simulink model "CalcTimes"  (R2024b)
settings: Solver=VariableStepAuto  StartTime=0.0  StopTime=10.0  RelTol=1e-3
settings Model: Creator=CArias  LastModifiedBy=CArias

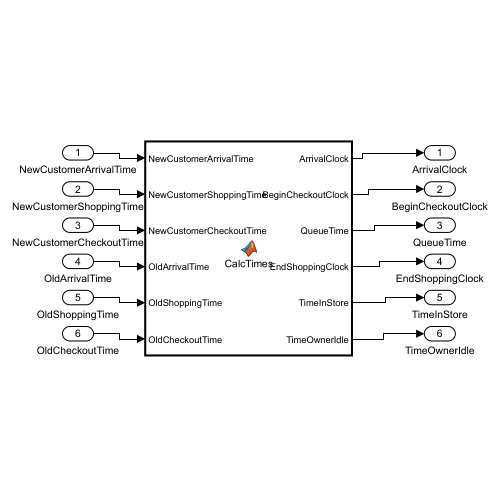
[thumbnail: Simulink's stored preview of the top-level diagram]
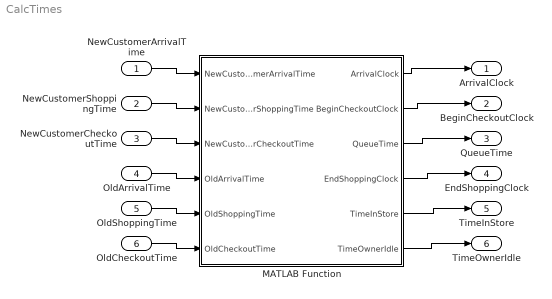
== system CalcTimes ==
  NewCustomerArrivalTime : Inport
  NewCustomerShoppingTime : Inport  Port=2
  NewCustomerCheckoutTime : Inport  Port=3
  OldArrivalTime : Inport  Port=4
  OldShoppingTime : Inport  Port=5
  OldCheckoutTime : Inport  Port=6
  MATLAB Function : MATLAB Function  TreatAsAtomicUnit=on
  ArrivalClock : Outport
  BeginCheckoutClock : Outport  Port=2
  QueueTime : Outport  Port=3
  EndShoppingClock : Outport  Port=4
  TimeInStore : Outport  Port=5
  TimeOwnerIdle : Outport  Port=6
  wires:
  NewCustomerArrivalTime/1 -> MATLAB Function/1(NewCustomerArrivalTime)
  NewCustomerShoppingTime/1 -> MATLAB Function/2(NewCustomerShoppingTime)
  NewCustomerCheckoutTime/1 -> MATLAB Function/3(NewCustomerCheckoutTime)
  OldArrivalTime/1 -> MATLAB Function/4(OldArrivalTime)
  OldShoppingTime/1 -> MATLAB Function/5(OldShoppingTime)
  OldCheckoutTime/1 -> MATLAB Function/6(OldCheckoutTime)
  MATLAB Function/1(ArrivalClock) -> ArrivalClock/1
  MATLAB Function/2(BeginCheckoutClock) -> BeginCheckoutClock/1
  MATLAB Function/3(QueueTime) -> QueueTime/1
  MATLAB Function/4(EndShoppingClock) -> EndShoppingClock/1
  MATLAB Function/5(TimeInStore) -> TimeInStore/1
  MATLAB Function/6(TimeOwnerIdle) -> TimeOwnerIdle/1

== matlab function CalcTimes/MATLAB Function ==
  data: NewCustomerArrivalTime input; ArrivalClock output; NewCustomerShoppingTime input; NewCustomerCheckoutTime input; OldArrivalTime input; OldShoppingTime input; OldCheckoutTime input; BeginCheckoutClock output; QueueTime output; EndShoppingClock output; TimeInStore output; TimeOwnerIdle output
function [ArrivalClock, BeginCheckoutClock, QueueTime, EndShoppingClock, TimeInStore, TimeOwnerIdle] = CalcTimes( ...
    NewCustomerArrivalTime, NewCustomerShoppingTime, NewCustomerCheckoutTime, ...
    OldArrivalTime, OldShoppingTime, OldCheckoutTime)

    % ArrivalClock is simply the time at which the new customer arrives
    ArrivalClock = OldArrivalTime + NewCustomerArrivalTime;
    
    % BeginCheckoutClock is the sum of ArrivalClock and the new customer's shopping time
    % the previous customer's EndShoppingClock and the new customer's BeginCheckoutClock
    PreviousEndShoppingClock = OldArrivalTime + OldShoppingTime + OldCheckoutTime;
    BeginCheckoutClock = max(PreviousEndShoppingClock, ArrivalClock + NewCustomerShoppingTime);
    
    % QueueTime is the waiting time in line; calculated as the difference between
    QueueTime = max(0, BeginCheckoutClock - PreviousEndShoppingClock);
    
    % EndShoppingClock is the time when the current customer finishes their checkout
    EndShoppingClock = BeginCheckoutClock + QueueTime + NewCustomerCheckoutTime;
    
    % TimeInStore is the total time the new customer spends in the store
    TimeInStore = EndShoppingClock - ArrivalClock;
    
    % TimeOwnerIdle is the idle time for the owner; calculated as the time between
    % the end of the previous customer's shopping and the new customer's BeginCheckoutClock
    TimeOwnerIdle = max(0, BeginCheckoutClock - PreviousEndShoppingClock);

end
